simulink model "landing"  (R2019a)
settings: Solver=VariableStepAuto  StartTime=0.0  StopTime=20  RelTol=1e-3  EnableMultiTasking=on
values from neighbouring files (symbols this model uses):
  A3 = zeros(5,5)    [Cesna182_flight_dy.m]
  B3 = [B1(:,1);zeros(1,1)]    [Cesna182_flight_dy.m]
  C3 = eye(5)    [Cesna182_flight_dy.m]
  D3 = zeros(5,1)    [Cesna182_flight_dy.m]
  K1 = K(:,1)    [Cesna182_flight_dy.m]
  Kx = K(:,2:end)    [Cesna182_flight_dy.m]
settings Model: Creator=-F.Machini  LastModifiedBy=yuril
settings DataIOCC: ReturnWorkspaceOutputs=off
settings OptimizationCC: LifeSpan=inf
settings DebuggingCC: SFUnexpectedBacktrackingDiag=warning  SFNoUnconditionalDefaultTransitionDiag=warning  ArithmeticOperatorsInVariantConditions=warning
settings SFSimCC: SimUseLocalCustomCode=off
settings RTWCC: RTWUseLocalCustomCode=off
settings CodeAppCC: StateflowObjectComments=on
settings GRTTargetCC: TargetLangStandard=C89/C90 (ANSI)  GeneratePreprocessorConditionals=Disable all
settings ConfigComp: CovMetricSettings=dw  CovHtmlReporting=on  CovSaveCumulativeToWorkspaceVar=on  CovSaveSingleToWorkspaceVar=on  CovExternalEMLEnable=off

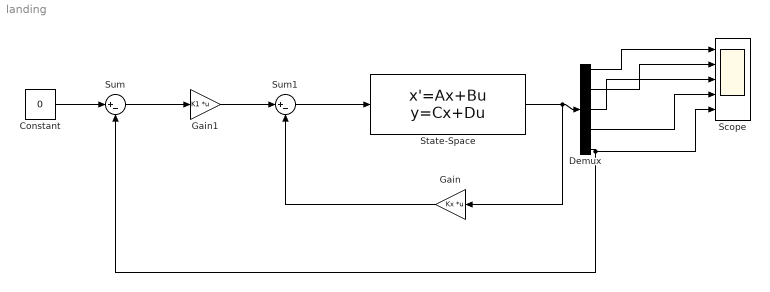
== system landing ==
  Constant : Constant  Value=0
  Demux : Demux  Outputs=5
  Gain : Gain  Gain=Kx  Multiplication=Matrix(K*u)
  Gain1 : Gain  Gain=K1  Multiplication=Matrix(K*u)
  Scope : Scope  NumInputPorts=5
  State-Space : StateSpace  A=A3  B=B3  C=C3  D=D3  InitialCondition=[0 0 0 0 100]
  Sum : Sum  Inputs=|+-
  Sum1 : Sum  Inputs=|+-
  wires:
  State-Space/1 -> Gain/1, Demux/1
  Demux/1 -> Scope/1
  Demux/3 -> Scope/3
  Demux/4 -> Scope/4
  Demux/2 -> Scope/2
  Gain1/1 -> Sum1/1
  Constant/1 -> Sum/1
  Sum/1 -> Gain1/1
  Sum1/1 -> State-Space/1
  Gain/1 -> Sum1/2
  Demux/5 -> Scope/5, Sum/2
